simulink model "ilc"  (Simulink 8.7)
settings: Solver=ode45  StartTime=0.0  StopTime=200  RelTol=1e-3
undefined symbols (not defined in the file): dt, gamma, Nseq
settings Model: Creator=aeagr  LastModifiedBy=aeagr
settings DataIOCC: SignalLoggingSaveFormat=ModelDataLogs
settings OptimizationCC: ExpressionDepthLimit=2147483647
settings DebuggingCC: SolverPrmCheckMsg=warning  FcnCallInpInsideContextMsg=EnableAllAsWarning  StateNameClashWarn=warning

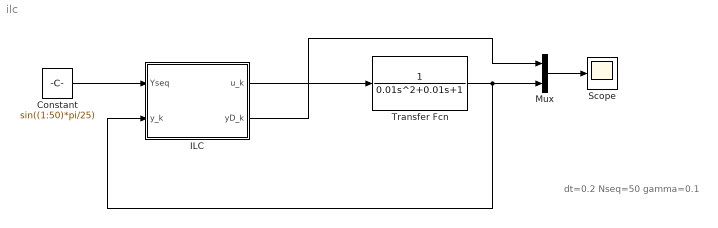
== system ilc ==
  note: dt=0.2
      | Nseq=50
      | gamma=0.1
  Constant : Constant  Value=sin((1:50)*pi/25)
  ILC : Subsystem  TreatAsAtomicUnit=on  SystemSampleTime=dt
  Mux : Mux  Inputs=2
  Scope : Scope
  Transfer Fcn : TransferFcn  Denominator=[0.01 0.01 1]
  wires:
  Transfer Fcn/1 -> ILC/2(y_k), Mux/2
  Constant/1 -> ILC/1(Yseq)
  ILC/2(yD_k) -> Mux/1
  Mux/1 -> Scope/1
  ILC/1(u_k) -> Transfer Fcn/1

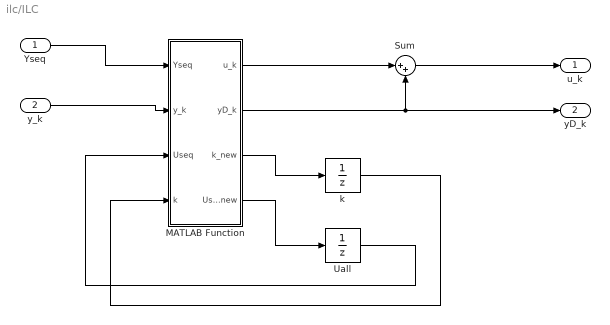
== system ilc/ILC ==
  Yseq : Inport
  y_k : Inport  Port=2
  MATLAB Function : MATLAB Function  TreatAsAtomicUnit=on
  Sum : Sum  Inputs=|++
  Uall : UnitDelay  InitialCondition=zeros(Nseq,1)  SampleTime=-1
  k : UnitDelay  InitialCondition=1  SampleTime=-1
  u_k : Outport
  yD_k : Outport  Port=2
  wires:
  MATLAB Function/3(k_new) -> k/1
  MATLAB Function/4(Useq_new) -> Uall/1
  Uall/1 -> MATLAB Function/3(Useq)
  y_k/1 -> MATLAB Function/2(y_k)
  Yseq/1 -> MATLAB Function/1(Yseq)
  k/1 -> MATLAB Function/4(k)
  MATLAB Function/2(yD_k) -> Sum/2, yD_k/1
  Sum/1 -> u_k/1
  MATLAB Function/1(u_k) -> Sum/1

== matlab function ILC/MATLAB Function ==
  data: u_k output double; Yseq input double; yD_k output double; y_k input double; Useq input double; k input double; Nseq parameter double; k_new output double; Useq_new output double; gamma parameter double
function [u_k,yD_k,k_new,Useq_new] = fcn(Yseq,y_k,Useq,k,Nseq,gamma)
%#codegen

% counter
k_new = k+1;
% reset if we've been round the sequence
if k_new>Nseq,
    k_new=1;
end

% extract current demand signal
yD_k = Yseq(k);

% and the current control
u_k = Useq(k);

% form the error
e_k = yD_k - y_k;

% copy the control sequence over
Useq_new = Useq;

% which entry to update
k_learn = k-1;
if k_learn<1,
    k_learn=Nseq;
end

% do the learning update
Useq_new(k_learn) = Useq_new(k_learn) + gamma*e_k;
